simulink model "Sim_Path_Forces"  (R2016a)
settings: Solver=VariableStepAuto  StartTime=0.0  StopTime=10.0  RelTol=1e-3
values from neighbouring files (symbols this model uses):
  ad = 0.1031    [alpha_equation.m]
  al = 0.8671    [alpha_equation.m]
  bd = 4.2706    [alpha_equation.m]
  bl = 7.1112    [alpha_equation.m]
undefined symbols (not defined in the file or in its folder): dynamic0
settings Model: Creator=Bakry  LastModifiedBy=Bakry

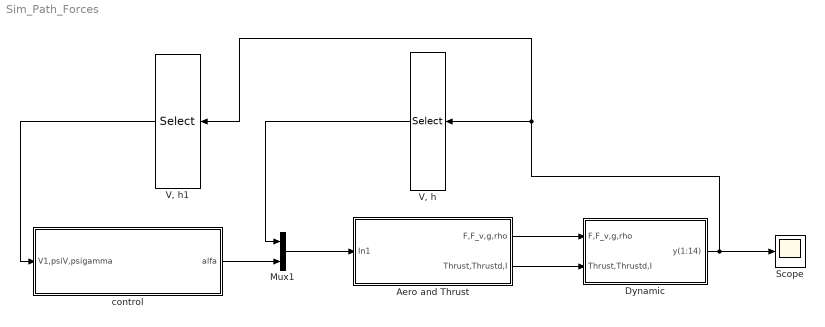
== system Sim_Path_Forces ==
  Aero and Thrust : Subsystem
  Dynamic : Subsystem
  Mux1 : Mux  Inputs=2
  Scope : Scope
  "V, h" : Selector  InputPortWidth=14  IndexOptions=Index vector (dialog)  Indices=[1 4]  OutputSizes=1
  "V, h1" : Selector  InputPortWidth=14  IndexOptions=Index vector (dialog)  Indices=[1 8 9]  OutputSizes=1
  control : Subsystem
  wires:
  Aero and Thrust/2(Thrust,Thrustd,I) -> Dynamic/2(Thrust,Thrustd,I)
  Aero and Thrust/1(F,F_v,g,rho) -> Dynamic/1(F,F_v,g,rho)
  Dynamic/1(y(1:14)) -> Scope/1, "V, h1"/1, "V, h"/1
  "V, h1"/1 -> control/1(V1,psiV,psigamma)
  Mux1/1 -> Aero and Thrust/1(In1)
  control/1(alfa) -> Mux1/2
  "V, h"/1 -> Mux1/1

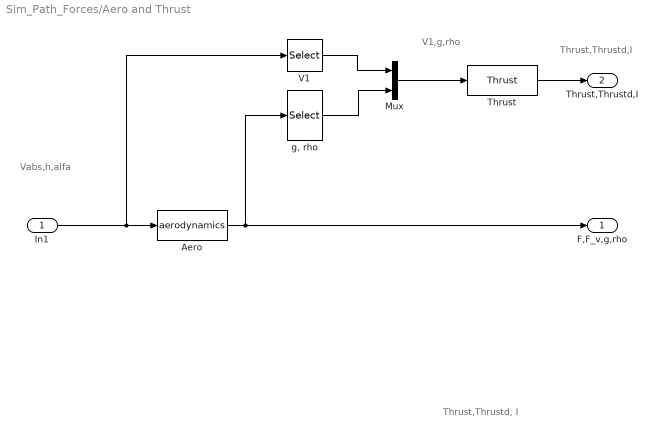
== system Sim_Path_Forces/Aero and Thrust ==
  note: Thrust,Thrustd,I
  note: Vabs,h,alfa
  note: Thrust,Thrustd, I
  note: V1,g,rho
  In1 : Inport
  Aero : MATLABFcn  MATLABFcn=aerodynamics  OutputDimensions=4
  Mux : Mux  Inputs=2
  Thrust : MATLABFcn  MATLABFcn=Thrust  OutputDimensions=3
  V1 : Selector  InputPortWidth=3  IndexOptions=Index vector (dialog)  Indices=[1]  OutputSizes=1
  "g, rho" : Selector  InputPortWidth=4  IndexOptions=Index vector (dialog)  Indices=[3 4]  OutputSizes=1
  F,F_v,g,rho : Outport
  Thrust,Thrustd,I : Outport  Port=2
  wires:
  Aero/1 -> "g, rho"/1, F,F_v,g,rho/1
  Mux/1 -> Thrust/1
  V1/1 -> Mux/1
  "g, rho"/1 -> Mux/2
  Thrust/1 -> Thrust,Thrustd,I/1
  In1/1 -> V1/1, Aero/1

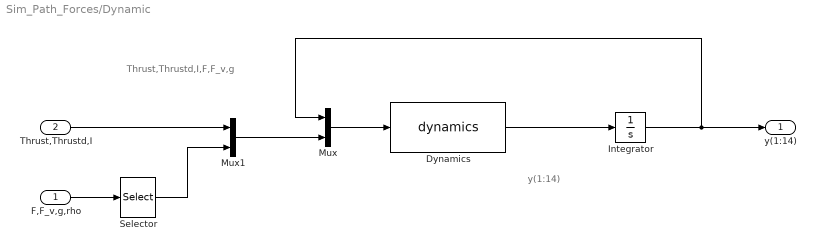
== system Sim_Path_Forces/Dynamic ==
  note: Thrust,Thrustd,I,F,F_v,g
  note: y(1:14)
  F,F_v,g,rho : Inport
  Thrust,Thrustd,I : Inport  Port=2
  Dynamics : MATLABFcn  MATLABFcn=dynamics  OutputDimensions=14
  Integrator : Integrator  InitialCondition=dynamic0
  Mux : Mux  Inputs=2
  Mux1 : Mux  Inputs=2
  Selector : Selector  InputPortWidth=4  IndexOptions=Index vector (dialog)  Indices=[1 2 3]  OutputSizes=1
  y(1:14) : Outport
  wires:
  Dynamics/1 -> Integrator/1
  Integrator/1 -> Mux/1, y(1:14)/1
  Mux/1 -> Dynamics/1
  Thrust,Thrustd,I/1 -> Mux1/1
  Mux1/1 -> Mux/2
  F,F_v,g,rho/1 -> Selector/1
  Selector/1 -> Mux1/2

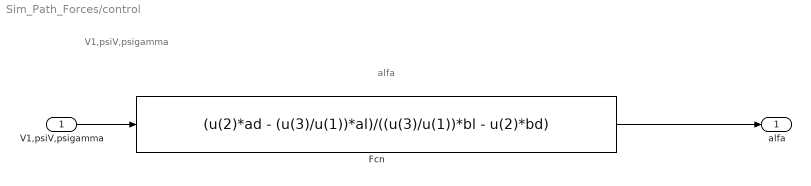
== system Sim_Path_Forces/control ==
  note: alfa
  note: V1,psiV,psigamma
  V1,psiV,psigamma : Inport
  Fcn : Fcn  Expr=(u(2)*ad - (u(3)/u(1))*al)/((u(3)/u(1))*bl - u(2)*bd)
  alfa : Outport
  wires:
  V1,psiV,psigamma/1 -> Fcn/1
  Fcn/1 -> alfa/1
